simulink model "TST_CrC_VD"  (R2016b)
settings: Solver=FixedStepDiscrete  StartTime=0.0  StopTime=simTime  FixedStep=sampleTime  RelTol=1e-3
values from neighbouring files (symbols this model uses):
  testCase = 1    [initTST_CrC_VD_001.m]    (also in initTST_CrC_VD_002.m = 2)
libraries: simulink x7, UnitTest_Lib x4
settings Model: Creator=xinchangran  LastModifiedBy=xinchangran
settings DebuggingCC: SignalRangeChecking=error

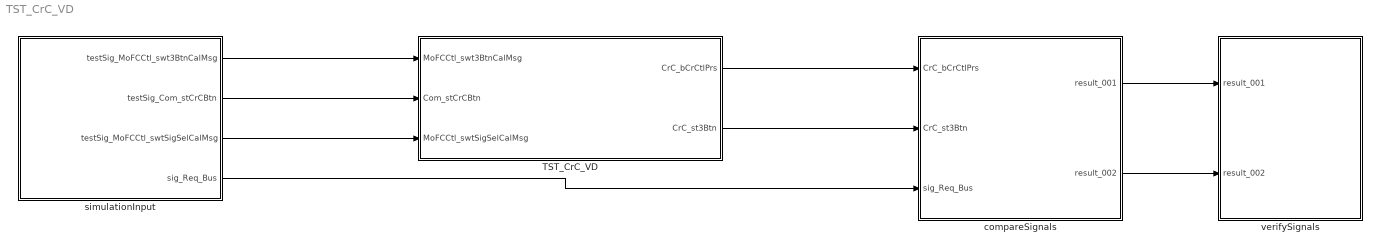
== system TST_CrC_VD ==
  TST_CrC_VD : Subsystem
  compareSignals : Subsystem
  simulationInput : Subsystem
  verifySignals : Subsystem
  wires:
  simulationInput/1(testSig_MoFCCtl_swt3BtnCalMsg) -> TST_CrC_VD/1(MoFCCtl_swt3BtnCalMsg)
  simulationInput/2(testSig_Com_stCrCBtn) -> TST_CrC_VD/2(Com_stCrCBtn)
  simulationInput/3(testSig_MoFCCtl_swtSigSelCalMsg) -> TST_CrC_VD/3(MoFCCtl_swtSigSelCalMsg)
  TST_CrC_VD/1(CrC_bCrCtlPrs) -> compareSignals/1(CrC_bCrCtlPrs)
  TST_CrC_VD/2(CrC_st3Btn) -> compareSignals/2(CrC_st3Btn)
  simulationInput/4(sig_Req_Bus) -> compareSignals/3(sig_Req_Bus)
  compareSignals/1(result_001) -> verifySignals/1(result_001)
  compareSignals/2(result_002) -> verifySignals/2(result_002)

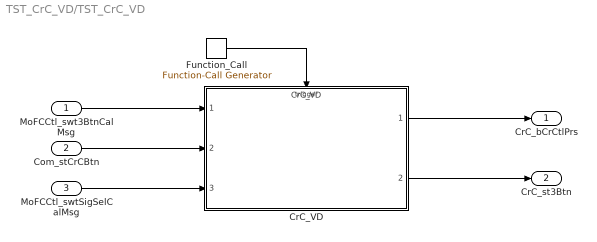
== system TST_CrC_VD/TST_CrC_VD ==
  MoFCCtl_swt3BtnCalMsg : Inport
  Com_stCrCBtn : Inport  Port=2
  MoFCCtl_swtSigSelCalMsg : Inport  Port=3
  CrC_VD : ModelReference  ModelNameDialog=CrC_VD  SimulationMode=Normal  ModelReferenceVersion=1.43  TriggerPortName=function  TriggerPortTriggerType=function-call  TriggerPortStatesWhenEnabling=held
  Function_Call : simulink/Ports & Subsystems/Function-Call Generator  sample_time=sampleTime  numberOfIterations=1
  CrC_bCrCtlPrs : Outport
  CrC_st3Btn : Outport  Port=2
  wires:
  Function_Call/1 -> CrC_VD/Trigger
  MoFCCtl_swt3BtnCalMsg/1 -> CrC_VD/1
  Com_stCrCBtn/1 -> CrC_VD/2
  MoFCCtl_swtSigSelCalMsg/1 -> CrC_VD/3
  CrC_VD/1 -> CrC_bCrCtlPrs/1
  CrC_VD/2 -> CrC_st3Btn/1

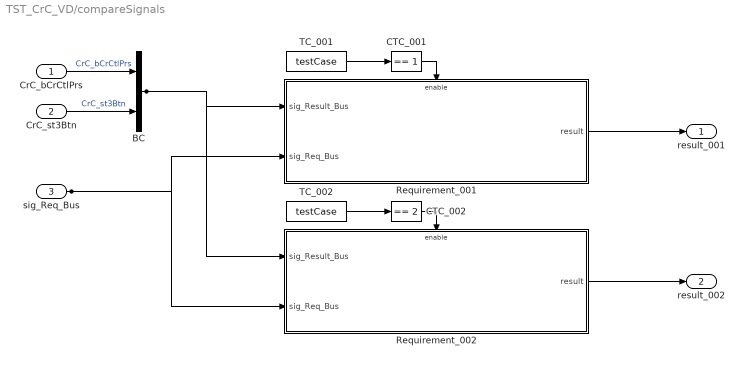
== system TST_CrC_VD/compareSignals ==
  CrC_bCrCtlPrs : Inport
  CrC_st3Btn : Inport  Port=2
  sig_Req_Bus : Inport  Port=3
  BC : BusCreator  Inputs=2
  CTC_001 : simulink/Logic and Bit Operations/Compare To Constant  relop===  const=1  OutDataTypeStr=boolean
  CTC_002 : simulink/Logic and Bit Operations/Compare To Constant  relop===  const=2  OutDataTypeStr=boolean
  Requirement_001 : Subsystem
  Requirement_002 : Subsystem
  TC_001 : Constant  Value=testCase
  TC_002 : Constant  Value=testCase
  result_001 : Outport
  result_002 : Outport  Port=2
  wires:
  CrC_bCrCtlPrs/1 -> BC/1  "CrC_bCrCtlPrs"
  CrC_st3Btn/1 -> BC/2  "CrC_st3Btn"
  TC_001/1 -> CTC_001/1
  CTC_001/1 -> Requirement_001/Enable
  sig_Req_Bus/1 -> Requirement_001/2(sig_Req_Bus), Requirement_002/2(sig_Req_Bus)
  BC/1 -> Requirement_001/1(sig_Result_Bus), Requirement_002/1(sig_Result_Bus)
  Requirement_001/1(result) -> result_001/1
  TC_002/1 -> CTC_002/1
  CTC_002/1 -> Requirement_002/Enable
  Requirement_002/1(result) -> result_002/1

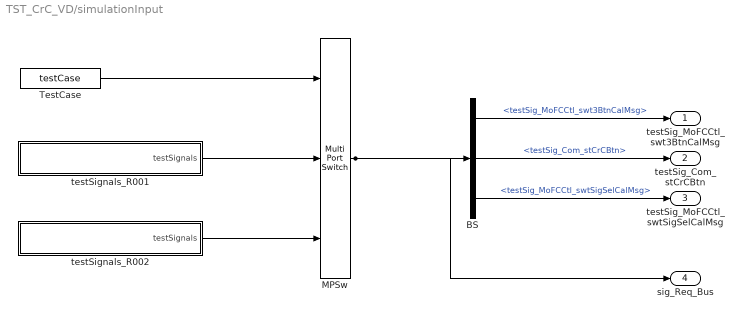
== system TST_CrC_VD/simulationInput ==
  BS : BusSelector  OutputSignals=testSig_MoFCCtl_swt3BtnCalMsg,testSig_Com_stCrCBtn,testSig_MoFCCtl_swtSigSelCalMsg
  MPSw : MultiPortSwitch  Inputs=2  SaturateOnIntegerOverflow=on  InputSameDT=on
  TestCase : Constant  Value=testCase
  testSignals_R001 : Subsystem
  testSignals_R002 : Subsystem
  testSig_MoFCCtl_swt3BtnCalMsg : Outport
  testSig_Com_stCrCBtn : Outport  Port=2
  testSig_MoFCCtl_swtSigSelCalMsg : Outport  Port=3
  sig_Req_Bus : Outport  Port=4
  wires:
  BS/1 -> testSig_MoFCCtl_swt3BtnCalMsg/1  "<testSig_MoFCCtl_swt3BtnCalMsg>"
  BS/2 -> testSig_Com_stCrCBtn/1  "<testSig_Com_stCrCBtn>"
  BS/3 -> testSig_MoFCCtl_swtSigSelCalMsg/1  "<testSig_MoFCCtl_swtSigSelCalMsg>"
  MPSw/1 -> BS/1, sig_Req_Bus/1
  TestCase/1 -> MPSw/1
  testSignals_R001/1(testSignals) -> MPSw/2
  testSignals_R002/1(testSignals) -> MPSw/3

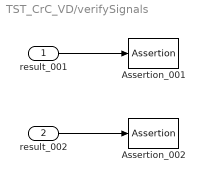
== system TST_CrC_VD/verifySignals ==
  result_001 : Inport
  result_002 : Inport  Port=2
  Assertion_001 : Assertion  Enabled=off
  Assertion_002 : Assertion  Enabled=off
  wires:
  result_001/1 -> Assertion_001/1
  result_002/1 -> Assertion_002/1

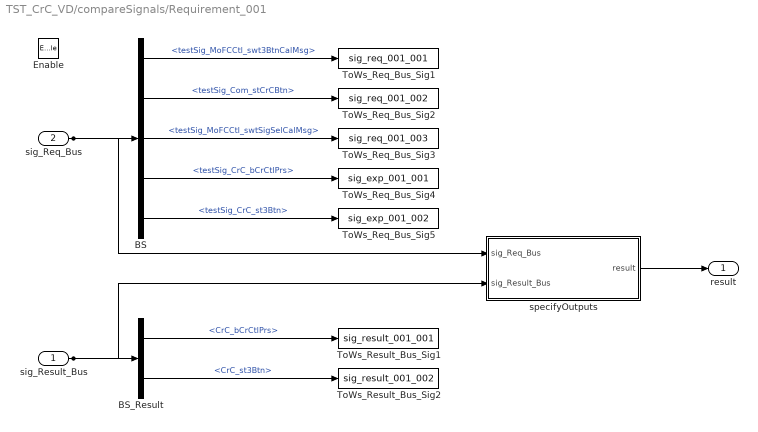
== system TST_CrC_VD/compareSignals/Requirement_001 ==
  sig_Result_Bus : Inport
  sig_Req_Bus : Inport  Port=2
  Enable : EnablePort
  BS : BusSelector  OutputSignals=testSig_MoFCCtl_swt3BtnCalMsg,testSig_Com_stCrCBtn,testSig_MoFCCtl_swtSigSelCalMsg,testSig_CrC_bCrCtlPrs,testSig_CrC_st3Btn
  BS_Result : BusSelector  OutputSignals=CrC_bCrCtlPrs,CrC_st3Btn
  ToWs_Req_Bus_Sig1 : ToWorkspace  VariableName=sig_req_001_001  SaveFormat=Structure With Time
  ToWs_Req_Bus_Sig2 : ToWorkspace  VariableName=sig_req_001_002  SaveFormat=Structure With Time
  ToWs_Req_Bus_Sig3 : ToWorkspace  VariableName=sig_req_001_003  SaveFormat=Structure With Time
  ToWs_Req_Bus_Sig4 : ToWorkspace  VariableName=sig_exp_001_001  SaveFormat=Structure With Time
  ToWs_Req_Bus_Sig5 : ToWorkspace  VariableName=sig_exp_001_002  SaveFormat=Structure With Time
  ToWs_Result_Bus_Sig1 : ToWorkspace  VariableName=sig_result_001_001  SaveFormat=Structure With Time
  ToWs_Result_Bus_Sig2 : ToWorkspace  VariableName=sig_result_001_002  SaveFormat=Structure With Time
  specifyOutputs : Subsystem
  result : Outport
  wires:
  sig_Req_Bus/1 -> BS/1, specifyOutputs/1(sig_Req_Bus)
  BS/1 -> ToWs_Req_Bus_Sig1/1  "<testSig_MoFCCtl_swt3BtnCalMsg>"
  BS/2 -> ToWs_Req_Bus_Sig2/1  "<testSig_Com_stCrCBtn>"
  BS/3 -> ToWs_Req_Bus_Sig3/1  "<testSig_MoFCCtl_swtSigSelCalMsg>"
  BS/4 -> ToWs_Req_Bus_Sig4/1  "<testSig_CrC_bCrCtlPrs>"
  BS/5 -> ToWs_Req_Bus_Sig5/1  "<testSig_CrC_st3Btn>"
  sig_Result_Bus/1 -> BS_Result/1, specifyOutputs/2(sig_Result_Bus)
  BS_Result/1 -> ToWs_Result_Bus_Sig1/1  "<CrC_bCrCtlPrs>"
  BS_Result/2 -> ToWs_Result_Bus_Sig2/1  "<CrC_st3Btn>"
  specifyOutputs/1(result) -> result/1

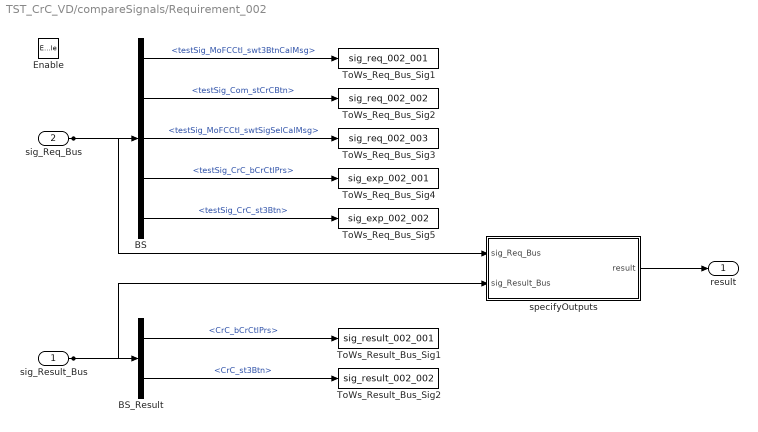
== system TST_CrC_VD/compareSignals/Requirement_002 ==
  sig_Result_Bus : Inport
  sig_Req_Bus : Inport  Port=2
  Enable : EnablePort
  BS : BusSelector  OutputSignals=testSig_MoFCCtl_swt3BtnCalMsg,testSig_Com_stCrCBtn,testSig_MoFCCtl_swtSigSelCalMsg,testSig_CrC_bCrCtlPrs,testSig_CrC_st3Btn
  BS_Result : BusSelector  OutputSignals=CrC_bCrCtlPrs,CrC_st3Btn
  ToWs_Req_Bus_Sig1 : ToWorkspace  VariableName=sig_req_002_001  SaveFormat=Structure With Time
  ToWs_Req_Bus_Sig2 : ToWorkspace  VariableName=sig_req_002_002  SaveFormat=Structure With Time
  ToWs_Req_Bus_Sig3 : ToWorkspace  VariableName=sig_req_002_003  SaveFormat=Structure With Time
  ToWs_Req_Bus_Sig4 : ToWorkspace  VariableName=sig_exp_002_001  SaveFormat=Structure With Time
  ToWs_Req_Bus_Sig5 : ToWorkspace  VariableName=sig_exp_002_002  SaveFormat=Structure With Time
  ToWs_Result_Bus_Sig1 : ToWorkspace  VariableName=sig_result_002_001  SaveFormat=Structure With Time
  ToWs_Result_Bus_Sig2 : ToWorkspace  VariableName=sig_result_002_002  SaveFormat=Structure With Time
  specifyOutputs : Subsystem
  result : Outport
  wires:
  sig_Req_Bus/1 -> BS/1, specifyOutputs/1(sig_Req_Bus)
  BS/1 -> ToWs_Req_Bus_Sig1/1  "<testSig_MoFCCtl_swt3BtnCalMsg>"
  BS/2 -> ToWs_Req_Bus_Sig2/1  "<testSig_Com_stCrCBtn>"
  BS/3 -> ToWs_Req_Bus_Sig3/1  "<testSig_MoFCCtl_swtSigSelCalMsg>"
  BS/4 -> ToWs_Req_Bus_Sig4/1  "<testSig_CrC_bCrCtlPrs>"
  BS/5 -> ToWs_Req_Bus_Sig5/1  "<testSig_CrC_st3Btn>"
  sig_Result_Bus/1 -> BS_Result/1, specifyOutputs/2(sig_Result_Bus)
  BS_Result/1 -> ToWs_Result_Bus_Sig1/1  "<CrC_bCrCtlPrs>"
  BS_Result/2 -> ToWs_Result_Bus_Sig2/1  "<CrC_st3Btn>"
  specifyOutputs/1(result) -> result/1

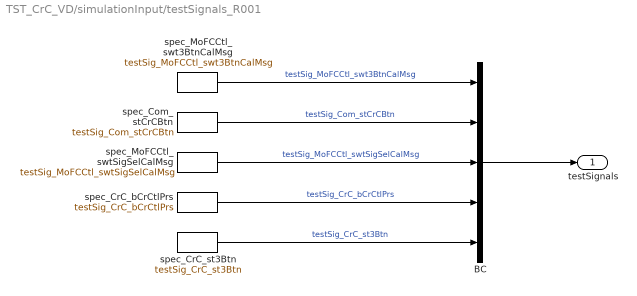
== system TST_CrC_VD/simulationInput/testSignals_R001 ==
  BC : BusCreator  Inputs=5
  spec_Com_stCrCBtn : FromWorkspace  VariableName=testSig_Com_stCrCBtn  Interpolate=off  OutputAfterFinalValue=Holding final value
  spec_CrC_bCrCtlPrs : FromWorkspace  VariableName=testSig_CrC_bCrCtlPrs  Interpolate=off  OutputAfterFinalValue=Holding final value
  spec_CrC_st3Btn : FromWorkspace  VariableName=testSig_CrC_st3Btn  Interpolate=off  OutputAfterFinalValue=Holding final value
  spec_MoFCCtl_swt3BtnCalMsg : FromWorkspace  VariableName=testSig_MoFCCtl_swt3BtnCalMsg  Interpolate=off  OutputAfterFinalValue=Holding final value
  spec_MoFCCtl_swtSigSelCalMsg : FromWorkspace  VariableName=testSig_MoFCCtl_swtSigSelCalMsg  Interpolate=off  OutputAfterFinalValue=Holding final value
  testSignals : Outport
  wires:
  BC/1 -> testSignals/1
  spec_MoFCCtl_swt3BtnCalMsg/1 -> BC/1  "testSig_MoFCCtl_swt3BtnCalMsg"
  spec_Com_stCrCBtn/1 -> BC/2  "testSig_Com_stCrCBtn"
  spec_MoFCCtl_swtSigSelCalMsg/1 -> BC/3  "testSig_MoFCCtl_swtSigSelCalMsg"
  spec_CrC_bCrCtlPrs/1 -> BC/4  "testSig_CrC_bCrCtlPrs"
  spec_CrC_st3Btn/1 -> BC/5  "testSig_CrC_st3Btn"

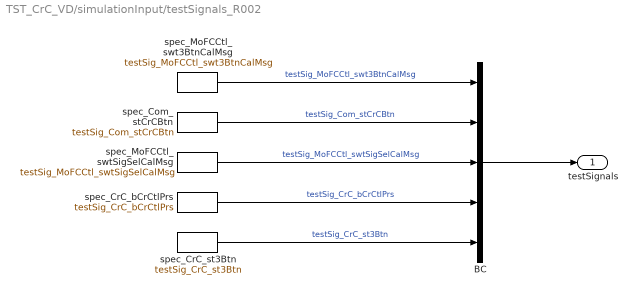
== system TST_CrC_VD/simulationInput/testSignals_R002 ==
  BC : BusCreator  Inputs=5
  spec_Com_stCrCBtn : FromWorkspace  VariableName=testSig_Com_stCrCBtn  Interpolate=off  OutputAfterFinalValue=Holding final value
  spec_CrC_bCrCtlPrs : FromWorkspace  VariableName=testSig_CrC_bCrCtlPrs  Interpolate=off  OutputAfterFinalValue=Holding final value
  spec_CrC_st3Btn : FromWorkspace  VariableName=testSig_CrC_st3Btn  Interpolate=off  OutputAfterFinalValue=Holding final value
  spec_MoFCCtl_swt3BtnCalMsg : FromWorkspace  VariableName=testSig_MoFCCtl_swt3BtnCalMsg  Interpolate=off  OutputAfterFinalValue=Holding final value
  spec_MoFCCtl_swtSigSelCalMsg : FromWorkspace  VariableName=testSig_MoFCCtl_swtSigSelCalMsg  Interpolate=off  OutputAfterFinalValue=Holding final value
  testSignals : Outport
  wires:
  BC/1 -> testSignals/1
  spec_MoFCCtl_swt3BtnCalMsg/1 -> BC/1  "testSig_MoFCCtl_swt3BtnCalMsg"
  spec_Com_stCrCBtn/1 -> BC/2  "testSig_Com_stCrCBtn"
  spec_MoFCCtl_swtSigSelCalMsg/1 -> BC/3  "testSig_MoFCCtl_swtSigSelCalMsg"
  spec_CrC_bCrCtlPrs/1 -> BC/4  "testSig_CrC_bCrCtlPrs"
  spec_CrC_st3Btn/1 -> BC/5  "testSig_CrC_st3Btn"

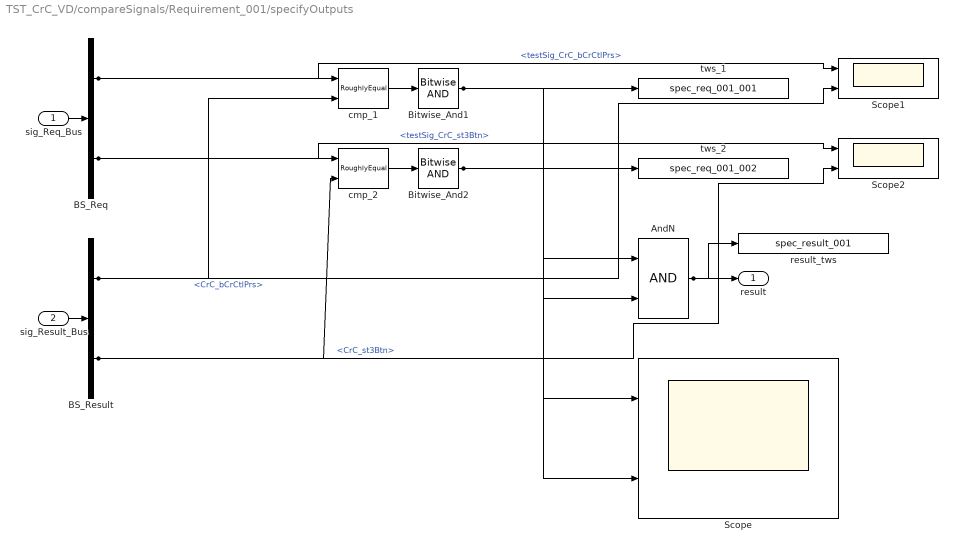
== system TST_CrC_VD/compareSignals/Requirement_001/specifyOutputs ==
  sig_Req_Bus : Inport
  sig_Result_Bus : Inport  Port=2
  AndN : Logic
  BS_Req : BusSelector  OutputSignals=testSig_CrC_bCrCtlPrs,testSig_CrC_st3Btn
  BS_Result : BusSelector  OutputSignals=CrC_bCrCtlPrs,CrC_st3Btn
  Bitwise_And1 : simulink/Logic and Bit Operations/Bitwise Operator  logicop=AND  UseBitMask=off  BitMask=bin2dec('11011001')  BitMaskRealWorld=Stored Integer
  Bitwise_And2 : simulink/Logic and Bit Operations/Bitwise Operator  logicop=AND  UseBitMask=off  BitMask=bin2dec('11011001')  BitMaskRealWorld=Stored Integer
  Scope : Scope  NumInputPorts=2
  Scope1 : Scope  NumInputPorts=2
  Scope2 : Scope  NumInputPorts=2
  cmp_1 : UnitTest_Lib/RoughlyEqual  slope=0.1
  cmp_2 : UnitTest_Lib/RoughlyEqual  slope=0.1
  result_tws : ToWorkspace  VariableName=spec_result_001
  tws_1 : ToWorkspace  VariableName=spec_req_001_001
  tws_2 : ToWorkspace  VariableName=spec_req_001_002
  result : Outport
  wires:
  sig_Req_Bus/1 -> BS_Req/1
  sig_Result_Bus/1 -> BS_Result/1
  AndN/1 -> result/1, result_tws/1
  BS_Req/1 -> cmp_1/1, Scope1/1  "<testSig_CrC_bCrCtlPrs>"
  BS_Result/1 -> cmp_1/2, Scope1/2  "<CrC_bCrCtlPrs>"
  cmp_1/1 -> Bitwise_And1/1
  Bitwise_And1/1 -> tws_1/1, AndN/1, Scope/1
  BS_Req/2 -> cmp_2/1, Scope2/1  "<testSig_CrC_st3Btn>"
  BS_Result/2 -> cmp_2/2, Scope2/2  "<CrC_st3Btn>"
  cmp_2/1 -> Bitwise_And2/1
  Bitwise_And2/1 -> tws_2/1, AndN/2, Scope/2

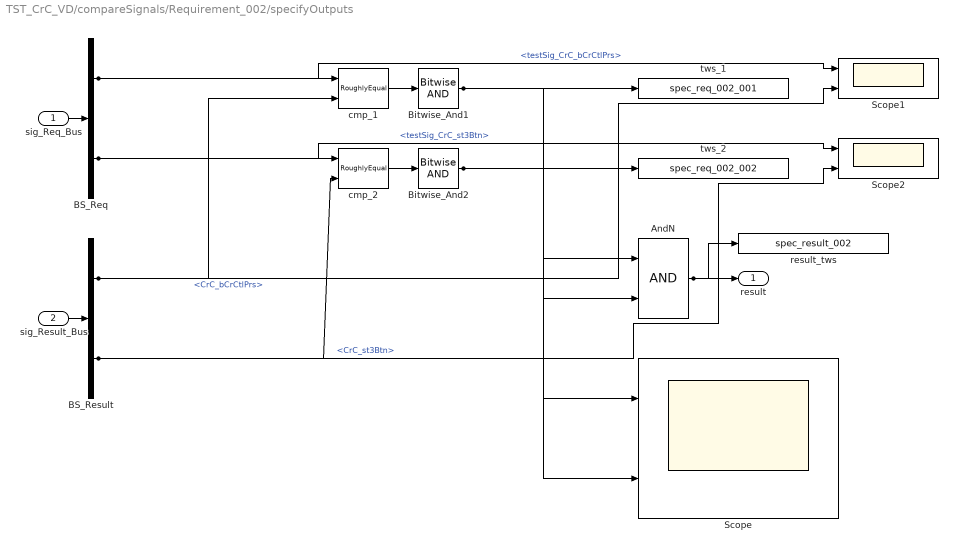
== system TST_CrC_VD/compareSignals/Requirement_002/specifyOutputs ==
  sig_Req_Bus : Inport
  sig_Result_Bus : Inport  Port=2
  AndN : Logic
  BS_Req : BusSelector  OutputSignals=testSig_CrC_bCrCtlPrs,testSig_CrC_st3Btn
  BS_Result : BusSelector  OutputSignals=CrC_bCrCtlPrs,CrC_st3Btn
  Bitwise_And1 : simulink/Logic and Bit Operations/Bitwise Operator  logicop=AND  UseBitMask=off  BitMask=bin2dec('11011001')  BitMaskRealWorld=Stored Integer
  Bitwise_And2 : simulink/Logic and Bit Operations/Bitwise Operator  logicop=AND  UseBitMask=off  BitMask=bin2dec('11011001')  BitMaskRealWorld=Stored Integer
  Scope : Scope  NumInputPorts=2
  Scope1 : Scope  NumInputPorts=2
  Scope2 : Scope  NumInputPorts=2
  cmp_1 : UnitTest_Lib/RoughlyEqual  slope=0.1
  cmp_2 : UnitTest_Lib/RoughlyEqual  slope=0.1
  result_tws : ToWorkspace  VariableName=spec_result_002
  tws_1 : ToWorkspace  VariableName=spec_req_002_001
  tws_2 : ToWorkspace  VariableName=spec_req_002_002
  result : Outport
  wires:
  sig_Req_Bus/1 -> BS_Req/1
  sig_Result_Bus/1 -> BS_Result/1
  AndN/1 -> result/1, result_tws/1
  BS_Req/1 -> cmp_1/1, Scope1/1  "<testSig_CrC_bCrCtlPrs>"
  BS_Result/1 -> cmp_1/2, Scope1/2  "<CrC_bCrCtlPrs>"
  cmp_1/1 -> Bitwise_And1/1
  Bitwise_And1/1 -> tws_1/1, AndN/1, Scope/1
  BS_Req/2 -> cmp_2/1, Scope2/1  "<testSig_CrC_st3Btn>"
  BS_Result/2 -> cmp_2/2, Scope2/2  "<CrC_st3Btn>"
  cmp_2/1 -> Bitwise_And2/1
  Bitwise_And2/1 -> tws_2/1, AndN/2, Scope/2
